simulink model "untitled"  (R2018a)
settings: Solver=VariableStepAuto  StartTime=0.0  StopTime=20  FixedStep=0.01  RelTol=1e-3
libraries: fuzblock x3
settings Model: Creator=kian  LastModifiedBy=Kasra

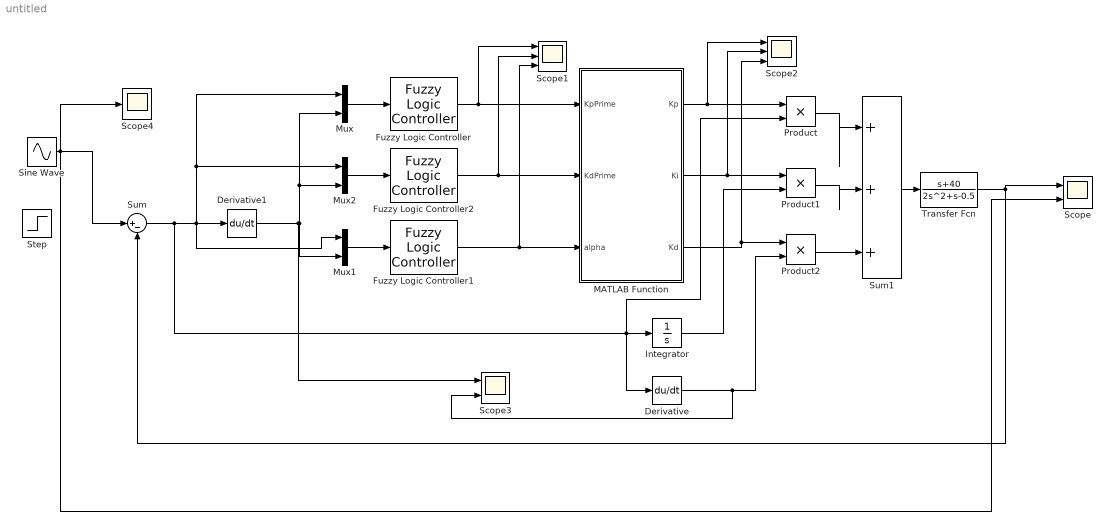
== system untitled ==
  Derivative : Derivative
  Derivative1 : Derivative
  Fuzzy Logic Controller : fuzblock/Fuzzy Logic  Controller  FIS='KpPrime.fis'  OutputSampleNumber=101  DataType=double  FuzzifiedInputs=off  RuleFiringStrengths=off  RuleOutputs=off  AggregatedOutputs=off  SimulateUsing=Interpreted execution  OutOfRangeInputValueMessage=warning  NoRuleFiredMessage=warning  EmptyOutputFuzzySetMessage=warning
  Fuzzy Logic Controller1 : fuzblock/Fuzzy Logic  Controller  FIS='alphaPrime.fis'  OutputSampleNumber=101  DataType=double  FuzzifiedInputs=off  RuleFiringStrengths=off  RuleOutputs=off  AggregatedOutputs=off  SimulateUsing=Interpreted execution  OutOfRangeInputValueMessage=warning  NoRuleFiredMessage=warning  EmptyOutputFuzzySetMessage=warning
  Fuzzy Logic Controller2 : fuzblock/Fuzzy Logic  Controller  FIS='KdPrime.fis'  OutputSampleNumber=101  DataType=double  FuzzifiedInputs=off  RuleFiringStrengths=off  RuleOutputs=off  AggregatedOutputs=off  SimulateUsing=Interpreted execution  OutOfRangeInputValueMessage=warning  NoRuleFiredMessage=warning  EmptyOutputFuzzySetMessage=warning
  Integrator : Integrator
  MATLAB Function : MATLAB Function  TreatAsAtomicUnit=on
  Mux : Mux  Inputs=2
  Mux1 : Mux  Inputs=2
  Mux2 : Mux  Inputs=2
  Product : Product
  Product1 : Product
  Product2 : Product
  Scope : Scope  NumInputPorts=2
  Scope1 : Scope  NumInputPorts=3
  Scope2 : Scope  NumInputPorts=3
  Scope3 : Scope  NumInputPorts=2
  Scope4 : Scope
  Sine Wave : Sin  SampleTime=0
  Step : Step  Time=0  SampleTime=0
  Sum : Sum  Inputs=|+-
  Sum1 : Sum  Inputs=|+++
  Transfer Fcn : TransferFcn  Numerator=[1 40]  Denominator=[2 1 -0.5]
  wires:
  Fuzzy Logic Controller/1 -> Scope1/1, MATLAB Function/1(KpPrime)
  Fuzzy Logic Controller2/1 -> Scope1/2, MATLAB Function/2(KdPrime)
  Fuzzy Logic Controller1/1 -> Scope1/3, MATLAB Function/3(alpha)
  Transfer Fcn/1 -> Scope/1, Sum/2
  Sum/1 -> Derivative/1, Product/2, Integrator/1, Derivative1/1, Mux/1, Mux2/1, Mux1/1
  Mux/1 -> Fuzzy Logic Controller/1
  Mux2/1 -> Fuzzy Logic Controller2/1
  Mux1/1 -> Fuzzy Logic Controller1/1
  Integrator/1 -> Product1/2
  Product2/1 -> Sum1/3
  Product1/1 -> Sum1/2
  Product/1 -> Sum1/1
  Sum1/1 -> Transfer Fcn/1
  Sine Wave/1 -> Sum/1, Scope/2, Scope4/1
  MATLAB Function/2(Ki) -> Product1/1, Scope2/2
  MATLAB Function/1(Kp) -> Scope2/1, Product/1
  MATLAB Function/3(Kd) -> Product2/1, Scope2/3
  Derivative1/1 -> Mux1/2, Mux/2, Mux2/2, Scope3/1
  Derivative/1 -> Scope3/2, Product2/2

== matlab function untitled/MATLAB Function ==
  data: KpPrime input; KdPrime input; alpha input; Kp output; Ki output; Kd output
function [Kp,Ki,Kd] = fcn(KpPrime,KdPrime, alpha)
kpmin = 0;
kpmax = 50;
Kp = KpPrime * (kpmax - kpmin) + kpmin;
kdmin = 0;
kdmax = 50;
Kd = KdPrime * (kdmax - kdmin) + kdmin;
Ki = (Kp * Kp)/(alpha * Kd);
